simulink model "Q4_Block_JM"  (R2021b)
settings: Solver=VariableStepAuto  StartTime=0.0  StopTime=10.0  RelTol=1e-3
libraries: cstblocks x8
settings Model: Creator=Bez  LastModifiedBy=Bez

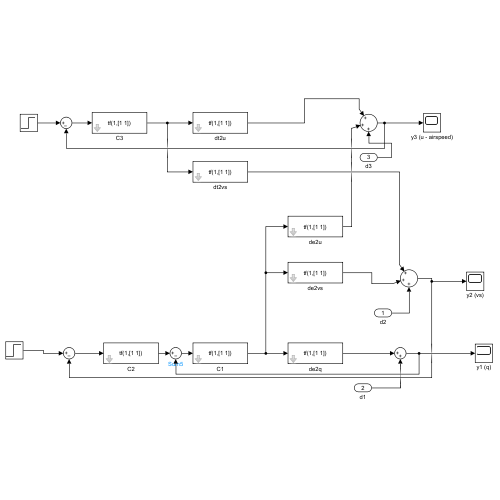
[thumbnail: Simulink's stored preview of the top-level diagram]
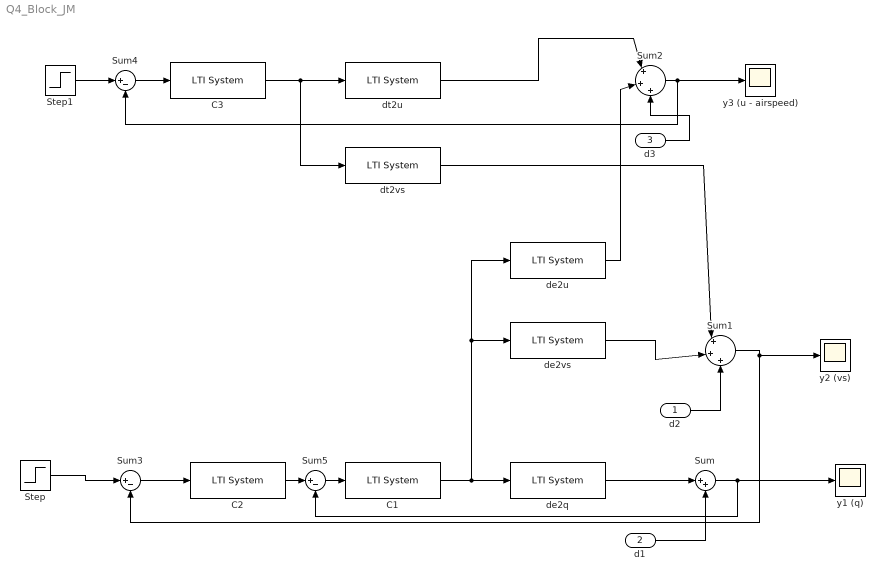
== system Q4_Block_JM ==
  d2 : Inport
  d1 : Inport  Port=2
  d3 : Inport  Port=3
  C1 : cstblocks/LTI System  sys=tf(1,[1 1])  IC=[]
  C2 : cstblocks/LTI System  sys=tf(1,[1 1])  IC=[]
  C3 : cstblocks/LTI System  sys=tf(1,[1 1])  IC=[]
  Step : Step  SampleTime=0
  Step1 : Step  SampleTime=0
  Sum : Sum  Inputs=|++
  Sum1 : Sum  Inputs=|+|+|+
  Sum2 : Sum  Inputs=|+|+|+
  Sum3 : Sum  Inputs=|+-
  Sum4 : Sum  Inputs=|+-
  Sum5 : Sum  Inputs=|+-
  de2q : cstblocks/LTI System  sys=tf(1,[1 1])  IC=[]
  de2u : cstblocks/LTI System  sys=tf(1,[1 1])  IC=[]
  de2vs : cstblocks/LTI System  sys=tf(1,[1 1])  IC=[]
  dt2u : cstblocks/LTI System  sys=tf(1,[1 1])  IC=[]
  dt2vs : cstblocks/LTI System  sys=tf(1,[1 1])  IC=[]
  y1 (q) : Scope
  y2 (vs) : Scope
  y3 (u - airspeed) : Scope
  wires:
  C3/1 -> dt2vs/1, dt2u/1
  dt2u/1 -> Sum2/1
  de2u/1 -> Sum2/2
  dt2vs/1 -> Sum1/1
  C1/1 -> de2u/1, de2vs/1, de2q/1
  de2vs/1 -> Sum1/2
  d2/1 -> Sum1/3
  de2q/1 -> Sum/1
  d1/1 -> Sum/2
  Sum3/1 -> C2/1
  Sum1/1 -> y2 (vs)/1, Sum3/2
  Step/1 -> Sum3/1
  d3/1 -> Sum2/3
  Sum2/1 -> y3 (u - airspeed)/1, Sum4/2
  Step1/1 -> Sum4/1
  Sum4/1 -> C3/1
  Sum/1 -> y1 (q)/1, Sum5/2
  C2/1 -> Sum5/1
  Sum5/1 -> C1/1
